simulink model "RegressFil_CodeGen_Interper_Different_Result"  (R2017b)
settings: Solver=VariableStepAuto  StartTime=0.0  StopTime=10.0  RelTol=1e-3
settings Model: Creator=81068  LastModifiedBy=81068

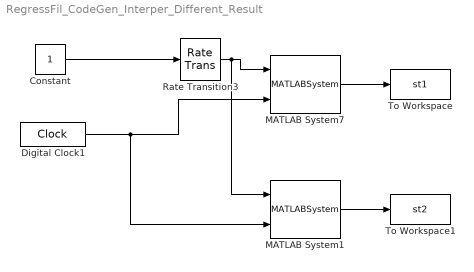
== system RegressFil_CodeGen_Interper_Different_Result ==
  Constant : Constant
  Digital Clock1 : DigitalClock  SampleTime=1/2000
  MATLAB System1 : MATLABSystem  System=JointFilter  sample_time=sample_time  history_length=history_length  dop=dop  signal_dim=1  SimulateUsing=Interpreted execution
      mask Type: JointFilter
      mask Display:
      | disp('JointFilter');
      | port_label('input',1,'q');
      | port_label('input',2,'t');
      | port_label('output',1,'dq');
  MATLAB System7 : MATLABSystem  System=JointFilter  sample_time=sample_time  history_length=history_length  dop=dop  signal_dim=1  SimulateUsing=Code generation
      mask Type: JointFilter
      mask Display:
      | disp('JointFilter');
      | port_label('input',1,'q');
      | port_label('input',2,'t');
      | port_label('output',1,'dq');
  Rate Transition3 : RateTransition  OutPortSampleTime=1/2000
  To Workspace : ToWorkspace  VariableName=st1  SaveFormat=Timeseries  SampleTime=-1
  To Workspace1 : ToWorkspace  VariableName=st2  SaveFormat=Timeseries  SampleTime=-1
  wires:
  Digital Clock1/1 -> MATLAB System1/2, MATLAB System7/2
  Constant/1 -> Rate Transition3/1
  MATLAB System7/1 -> To Workspace/1
  MATLAB System1/1 -> To Workspace1/1
  Rate Transition3/1 -> MATLAB System1/1, MATLAB System7/1
